simulink model "Two_mass_stifness_system_modal_controller"  (R2013b)
settings: Solver=ode3  StartTime=0.0  StopTime=2  FixedStep=1e-5  RelTol=1e-3
values from neighbouring files (symbols this model uses):
  c = GJp/l    (= 0.0104)    [params.m]
  ce = (Un - In*R)/wn    (= 0.301701587302)    [params.m]
  cm = Mn/In    (= 0.212068965517)    [params.m]
  Jadd = Jm/10    (= 5.9e-06)    [params.m]
  Jm = 0.59*10^(-4)    (= 5.9e-05)    [params.m]
  K = place(A,B,p)    [script.m]
  Mn = 0.123    [params.m]
  R = 25.8    [params.m]
undefined symbols (not defined in the file or in its folder): A, B, C
settings Model: Creator=user  LastModifiedBy=user
settings DataIOCC: LimitDataPoints=off  OutputSaveName=out1

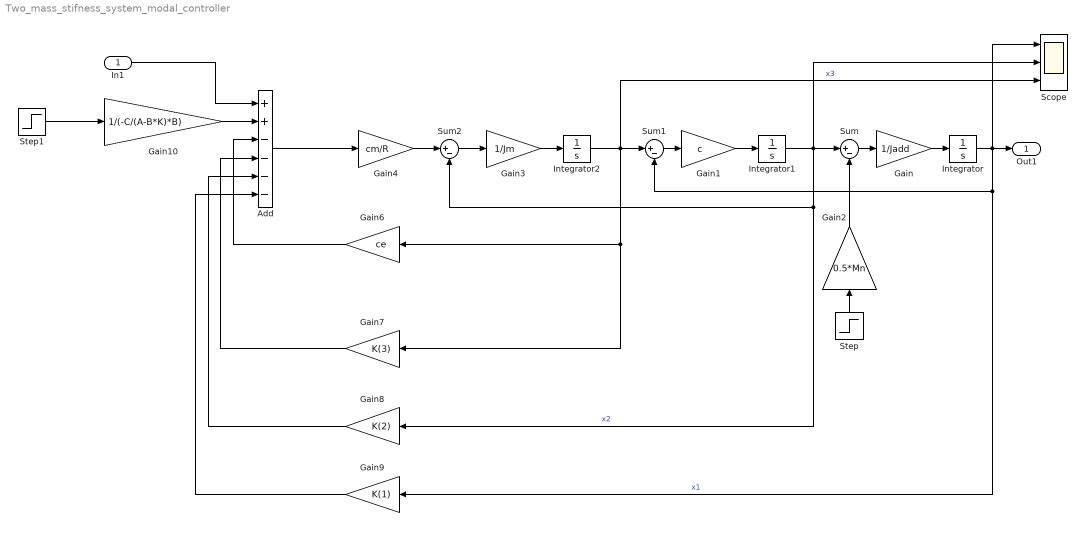
== system Two_mass_stifness_system_modal_controller ==
  In1 : Inport
  Add : Sum  Inputs=++----
  Gain : Gain  Gain=1/Jadd
  Gain1 : Gain  Gain=c
  Gain10 : Gain  Gain=1/(-C/(A-B*K)*B)
  Gain2 : Gain  Gain=0.5*Mn
  Gain3 : Gain  Gain=1/Jm
  Gain4 : Gain  Gain=cm/R
  Gain6 : Gain  Gain=ce
  Gain7 : Gain  Gain=K(3)
  Gain8 : Gain  Gain=K(2)
  Gain9 : Gain  Gain=K(1)
  Integrator : Integrator
  Integrator1 : Integrator
  Integrator2 : Integrator
  Scope : Scope  NumInputPorts=3
      settings: YMin=-5~-5~-5  YMax=5~5~5
  Step : Step  Time=0  SampleTime=0
  Step1 : Step  Time=0  SampleTime=0
  Sum : Sum  Inputs=|+-
  Sum1 : Sum  Inputs=|+-
  Sum2 : Sum  Inputs=|+-
  Out1 : Outport
  wires:
  Sum/1 -> Gain/1
  Gain/1 -> Integrator/1
  Gain1/1 -> Integrator1/1
  Integrator1/1 -> Gain8/1, Sum2/2, Scope/2, Sum/1  "x2"
  Sum1/1 -> Gain1/1
  Integrator/1 -> Gain9/1, Sum1/2, Scope/1, Out1/1  "x1"
  Gain3/1 -> Integrator2/1
  Integrator2/1 -> Gain7/1, Gain6/1, Scope/3, Sum1/1  "x3"
  Sum2/1 -> Gain3/1
  Gain4/1 -> Sum2/1
  Gain6/1 -> Add/3
  Step/1 -> Gain2/1
  Add/1 -> Gain4/1
  In1/1 -> Add/1
  Gain2/1 -> Sum/2
  Step1/1 -> Gain10/1
  Gain10/1 -> Add/2
  Gain7/1 -> Add/4
  Gain8/1 -> Add/5
  Gain9/1 -> Add/6
